simulink model "testingarx"  (R2024a)
settings: Solver=FixedStepAuto  StartTime=0.0  StopTime=100  FixedStep=1  RelTol=1e-3
libraries: simulink x1
settings Model: Creator=hp  LastModifiedBy=hp

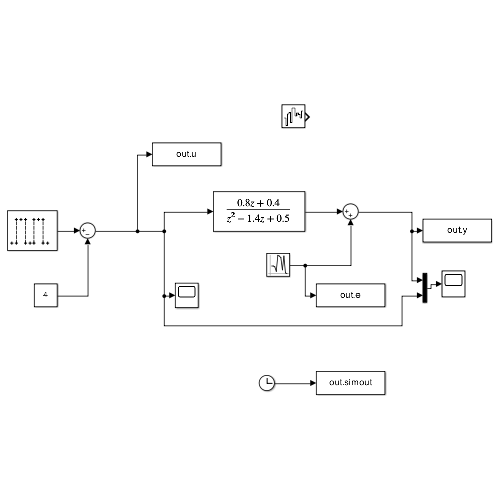
[thumbnail: Simulink's stored preview of the top-level diagram]
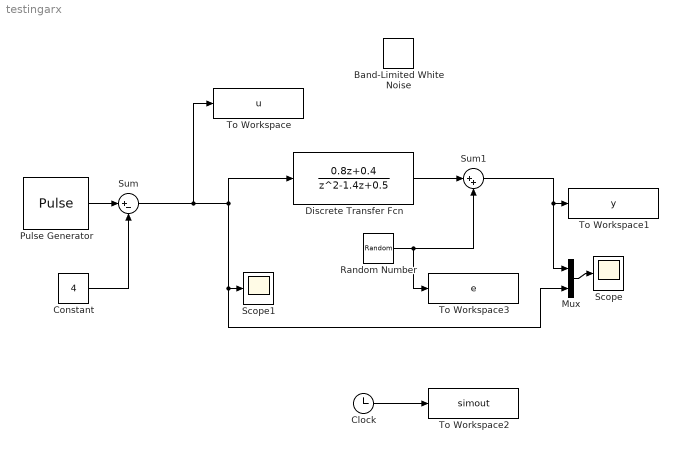
== system testingarx ==
  Band-Limited White Noise : simulink/Sources/Band-Limited White Noise  Cov=[0.1]  Ts=1  seed=[23341]
  Clock : Clock
  Constant : Constant  Value=4
  Discrete Transfer Fcn : DiscreteTransferFcn  Numerator=[0.8 0.4]  Denominator=[1 -1.4 0.5]
  Mux : Mux  Inputs=2
  Pulse Generator : DiscretePulseGenerator  Amplitude=8  Period=50  PulseWidth=25
  Random Number : RandomNumber  Variance=0.1  Seed=23341  SampleTime=1
  Scope : Scope
  Scope1 : Scope
  Sum : Sum  Inputs=|+-
  Sum1 : Sum  Inputs=|++
  To Workspace : ToWorkspace  VariableName=u  SaveFormat=Timeseries  SampleTime=-1
  To Workspace1 : ToWorkspace  VariableName=y  SaveFormat=Timeseries  SampleTime=-1
  To Workspace2 : ToWorkspace  VariableName=simout  SaveFormat=Timeseries  SampleTime=-1
  To Workspace3 : ToWorkspace  VariableName=e  SaveFormat=Timeseries  SampleTime=-1
  wires:
  Sum/1 -> Discrete Transfer Fcn/1, Mux/2, Scope1/1, To Workspace/1
  Sum1/1 -> Mux/1, To Workspace1/1
  Clock/1 -> To Workspace2/1
  Mux/1 -> Scope/1
  Random Number/1 -> To Workspace3/1, Sum1/2
  Pulse Generator/1 -> Sum/1
  Constant/1 -> Sum/2
  Discrete Transfer Fcn/1 -> Sum1/1
